simulink model "controller2"  (R2024b)
settings: Solver=FixedStepAuto  StartTime=0.0  StopTime=9  FixedStep=0.05  RelTol=1e-3
model workspace (MAT data in the model file):
  SamplePd = 0.05
values from neighbouring files (symbols this model uses):
  DryMass = 3    [FlightPathGeneration.m]
  LaunchSitePressure = PlanMeta(7)    [FlightAnalysis.m]    (also in FlightPathGeneration.m = 101325; TargetApogeeSelection.m = 101325)
  LaunchSiteTemperature = PlanMeta(6)    [FlightAnalysis.m]    (also in FlightPathGeneration.m = 288.15; TargetApogeeSelection.m = 288.15)
  MaximumDragArea = 0.01    [FlightPathGeneration.m]    (also in TargetApogeeSelection.m)
  MinimumDragArea = 0.0025    [FlightPathGeneration.m]    (also in TargetApogeeSelection.m)
  SimAngleSamples = linspace(0, pi/2, AngleSamples)    [FlightPathGeneration.m]
  SimGradAngleMesh = SimGradAngleMesh(end:-1:1, end:-1:1)'    [FlightPathGeneration.m]
  SimGradVMesh = SimGradVMesh(end:-1:1, end:-1:1)'    [FlightPathGeneration.m]
  SimMesh = centerPathAltitudes(end:-1:1, end:-1:1)'    [FlightPathGeneration.m]
  SimVelocitySamples = linspace(0, MaxVelocity, VelocitySamples)    [FlightPathGeneration.m]
undefined symbols (not defined in the file or in its folder): DiscIntNeverNeededParam
settings Model: Creator=natha  LastModifiedBy=natha

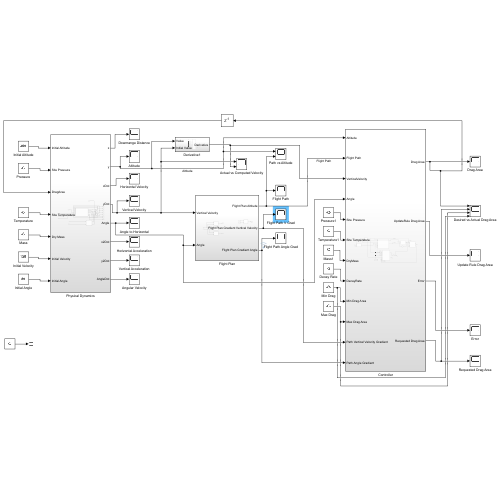
[thumbnail: Simulink's stored preview of the top-level diagram]
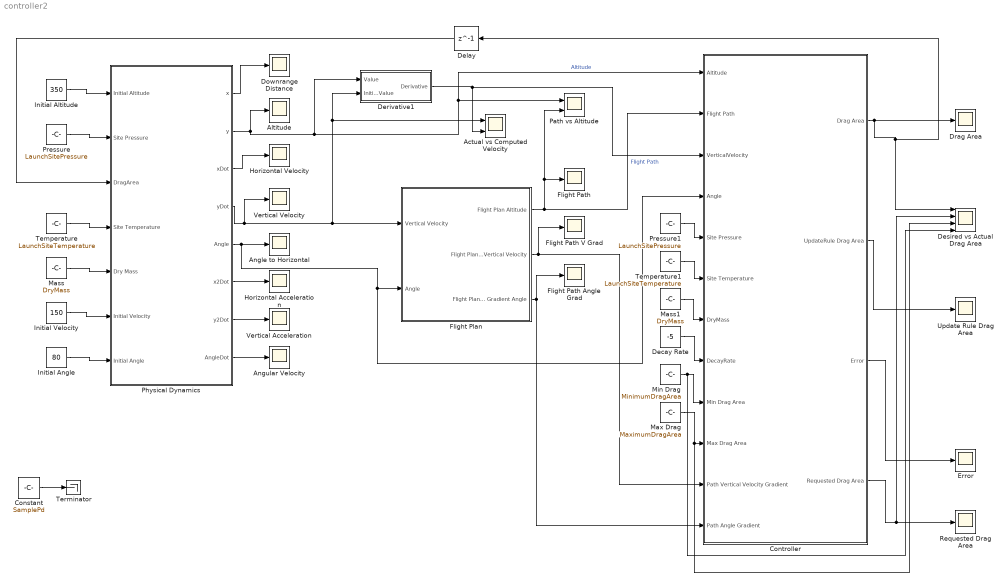
== system controller2 ==
  Actual vs Computed Velocity : Scope  NumInputPorts=2
  Altitude : Scope
  Angle to Horizontal : Scope
  Angular Velocity : Scope
  Constant : Constant  Value=SamplePd
  Controller : Subsystem
  Decay Rate : Constant  Value=-5
  Delay : Delay  DelayLength=1  InputProcessing=Columns as channels (frame based)
  Derivative1 : Subsystem
  Desired vs Actual Drag Area : Scope  NumInputPorts=4
  Downrange Distance : Scope
  Drag Area : Scope
  Error : Scope
  Flight Path : Scope
  Flight Path Angle Grad : Scope
  Flight Path V Grad : Scope
  Flight Plan : Subsystem
  Horizontal Acceleration : Scope
  Horizontal Velocity : Scope
  Initial Altitude : Constant  Value=350
  Initial Angle : Constant  Value=80
  Initial Velocity : Constant  Value=150
  Mass : Constant  Value=DryMass
  Mass1 : Constant  Value=DryMass
  Max Drag : Constant  Value=MaximumDragArea
  Min Drag : Constant  Value=MinimumDragArea
  Path vs Altitude : Scope  NumInputPorts=2
  Physical Dynamics : Subsystem
  Pressure : Constant  Value=LaunchSitePressure
  Pressure1 : Constant  Value=LaunchSitePressure
  Requested Drag Area : Scope
  Temperature : Constant  Value=LaunchSiteTemperature
  Temperature1 : Constant  Value=LaunchSiteTemperature
  Terminator : Terminator
  Update Rule Drag Area : Scope
  Vertical Acceleration : Scope
  Vertical Velocity : Scope
  wires:
  Initial Altitude/1 -> Physical Dynamics/1(Initial Altitude)
  Pressure/1 -> Physical Dynamics/2(Site Pressure)
  Temperature/1 -> Physical Dynamics/4(Site Temperature)
  Mass/1 -> Physical Dynamics/5(Dry Mass)
  Initial Velocity/1 -> Physical Dynamics/6(Initial Velocity)
  Initial Angle/1 -> Physical Dynamics/7(Initial Angle)
  Physical Dynamics/1(x) -> Downrange Distance/1
  Physical Dynamics/2(y) -> Derivative1/1(Value), Controller/1(Altitude), Path vs Altitude/1, Altitude/1  "Altitude"
  Physical Dynamics/3(xDot) -> Horizontal Velocity/1
  Physical Dynamics/4(yDot) -> Actual vs Computed Velocity/1, Derivative1/2(Initial Value), Flight Plan/1(Vertical Velocity), Vertical Velocity/1
  Physical Dynamics/5(Angle) -> Controller/4(Angle), Flight Plan/2(Angle), Angle to Horizontal/1
  Physical Dynamics/7(y2Dot) -> Vertical Acceleration/1
  Physical Dynamics/6(x2Dot) -> Horizontal Acceleration/1
  Flight Plan/1(Flight Plan Altitude) -> Controller/2(Flight Path), Path vs Altitude/2, Flight Path/1  "Flight Path"
  Flight Plan/2(Flight Plan Gradient Vertical Velocity) -> Controller/11(Path Vertical Velocity Gradient), Flight Path V Grad/1
  Flight Plan/3(Flight Plan Gradient Angle) -> Controller/12(Path Angle Gradient), Flight Path Angle Grad/1
  Min Drag/1 -> Desired vs Actual Drag Area/4, Controller/9(Min Drag Area)
  Max Drag/1 -> Desired vs Actual Drag Area/3, Controller/10(Max Drag Area)
  Decay Rate/1 -> Controller/8(DecayRate)
  Temperature1/1 -> Controller/6(Site Temperature)
  Pressure1/1 -> Controller/5(Site Pressure)
  Mass1/1 -> Controller/7(DryMass)
  Physical Dynamics/8(AngleDot) -> Angular Velocity/1
  Controller/2(UpdateRule Drag Area) -> Update Rule Drag Area/1
  Controller/1(Drag Area) -> Delay/1, Desired vs Actual Drag Area/1, Drag Area/1
  Controller/3(Error) -> Error/1
  Delay/1 -> Physical Dynamics/3(DragArea)
  Constant/1 -> Terminator/1
  Derivative1/1(Derivative) -> Controller/3(VerticalVelocity), Actual vs Computed Velocity/2
  Controller/4(Requested Drag Area) -> Desired vs Actual Drag Area/2, Requested Drag Area/1

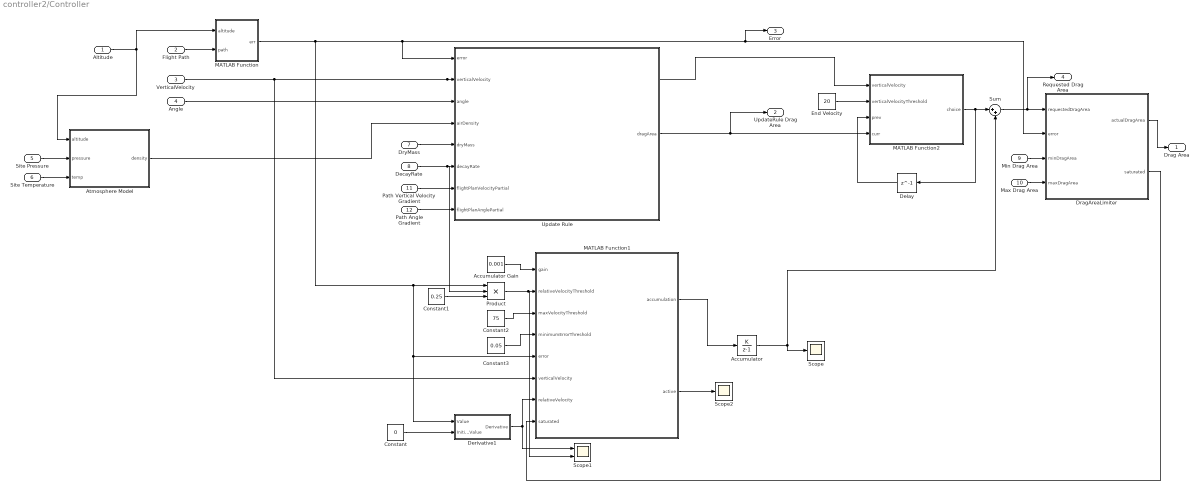
== system controller2/Controller ==
  Altitude : Inport
  Flight Path : Inport  Port=2
  VerticalVelocity : Inport  Port=3
  Angle : Inport  Port=4
  Site Pressure : Inport  Port=5
  Site Temperature : Inport  Port=6
  DryMass : Inport  Port=7
  DecayRate : Inport  Port=8
  Min Drag Area : Inport  Port=9
  Max Drag Area : Inport  Port=10
  Path Vertical Velocity Gradient : Inport  Port=11
  Path Angle Gradient : Inport  Port=12
  Accumulator : DiscreteIntegrator  IntegratorMethod=Accumulation: Forward Euler  SampleTime=-1  ICPrevOutput=DiscIntNeverNeededParam  ICPrevScaledInput=DiscIntNeverNeededParam
  Accumulator Gain : Constant  Value=0.001
  Atmosphere Model : MATLAB Function  TreatAsAtomicUnit=on
  Constant : Constant  Value=0
  Constant1 : Constant  Value=0.25
  Constant2 : Constant  Value=75
  Constant3 : Constant  Value=0.05
  Delay : Delay  DelayLength=1  InputProcessing=Columns as channels (frame based)
  Derivative1 : Subsystem
  DragAreaLimiter : MATLAB Function  TreatAsAtomicUnit=on
  End Velocity : Constant  Value=20
  MATLAB Function : MATLAB Function  TreatAsAtomicUnit=on
  MATLAB Function1 : MATLAB Function  TreatAsAtomicUnit=on
  MATLAB Function2 : MATLAB Function  TreatAsAtomicUnit=on
  Product : Product  Inputs=3
  Scope : Scope
  Scope1 : Scope  NumInputPorts=2
  Scope2 : Scope
  Sum : Sum  Inputs=|++
  Update Rule : MATLAB Function  TreatAsAtomicUnit=on
  Drag Area : Outport
  UpdateRule Drag Area : Outport  Port=2
  Error : Outport  Port=3
  Requested Drag Area : Outport  Port=4
  wires:
  DecayRate/1 -> Update Rule/6(decayRate), Product/2
  Max Drag Area/1 -> DragAreaLimiter/4(maxDragArea)
  DryMass/1 -> Update Rule/5(dryMass)
  Min Drag Area/1 -> DragAreaLimiter/3(minDragArea)
  Update Rule/1(dragArea) -> MATLAB Function2/4(curr), UpdateRule Drag Area/1
  Atmosphere Model/1(density) -> Update Rule/4(airDensity)
  Altitude/1 -> Atmosphere Model/1(altitude), MATLAB Function/1(altitude)
  MATLAB Function/1(err) -> Derivative1/1(Value), MATLAB Function1/5(error), Product/1, Update Rule/1(error), DragAreaLimiter/2(error), Error/1
  Site Temperature/1 -> Atmosphere Model/3(temp)
  Site Pressure/1 -> Atmosphere Model/2(pressure)
  Flight Path/1 -> MATLAB Function/2(path)
  Angle/1 -> Update Rule/3(angle)
  Path Angle Gradient/1 -> Update Rule/8(flightPlanAnglePartial)
  VerticalVelocity/1 -> MATLAB Function1/6(verticalVelocity), MATLAB Function2/1(verticalVelocity), Update Rule/2(verticalVelocity)
  Path Vertical Velocity Gradient/1 -> Update Rule/7(flightPlanVelocityPartial)
  MATLAB Function1/1(accumulation) -> Accumulator/1
  Accumulator Gain/1 -> MATLAB Function1/1(gain)
  Constant2/1 -> MATLAB Function1/3(maxVelocityThreshold)
  Constant3/1 -> MATLAB Function1/4(minimumErrorThreshold)
  Constant1/1 -> Product/3
  Product/1 -> Scope1/2, MATLAB Function1/2(relativeVelocityThreshold)
  Derivative1/1(Derivative) -> Scope1/1, MATLAB Function1/7(relativeVelocity)
  Constant/1 -> Derivative1/2(Initial Value)
  Accumulator/1 -> Sum/2, Scope/1
  MATLAB Function1/2(active) -> Scope2/1
  MATLAB Function2/1(choice) -> Sum/1, Delay/1
  Delay/1 -> MATLAB Function2/3(prev)
  End Velocity/1 -> MATLAB Function2/2(verticalVelocityThreshold)
  Sum/1 -> Requested Drag Area/1, DragAreaLimiter/1(requestedDragArea)
  DragAreaLimiter/1(actualDragArea) -> Drag Area/1
  DragAreaLimiter/2(saturated) -> MATLAB Function1/8(saturated)

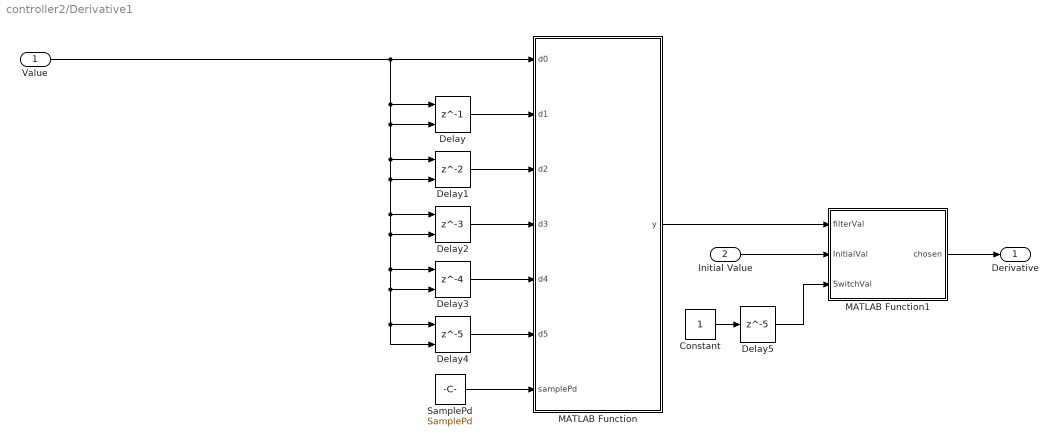
== system controller2/Derivative1 ==
  Value : Inport
  Initial Value : Inport  Port=2
  Constant : Constant
  Delay : Delay  DelayLength=1  InitialConditionSource=Input port  InputProcessing=Columns as channels (frame based)
      settings: InputPortMap=u0,p4
  Delay1 : Delay  InitialConditionSource=Input port  InputProcessing=Columns as channels (frame based)
      settings: InputPortMap=u0,p4
  Delay2 : Delay  DelayLength=3  InitialConditionSource=Input port  InputProcessing=Columns as channels (frame based)
      settings: InputPortMap=u0,p4
  Delay3 : Delay  DelayLength=4  InitialConditionSource=Input port  InputProcessing=Columns as channels (frame based)
      settings: InputPortMap=u0,p4
  Delay4 : Delay  DelayLength=5  InitialConditionSource=Input port  InputProcessing=Columns as channels (frame based)
      settings: InputPortMap=u0,p4
  Delay5 : Delay  DelayLength=5  InputProcessing=Columns as channels (frame based)
  MATLAB Function : MATLAB Function  TreatAsAtomicUnit=on
  MATLAB Function1 : MATLAB Function  TreatAsAtomicUnit=on
  SamplePd : Constant  Value=SamplePd
  Derivative : Outport
  wires:
  Value/1 -> Delay2/2, Delay3/2, Delay4/2, Delay4/1, Delay3/1, Delay2/1, Delay1/2, Delay1/1, Delay/2, Delay/1, MATLAB Function/1(d0)
  Delay/1 -> MATLAB Function/2(d1)
  Delay1/1 -> MATLAB Function/3(d2)
  Delay2/1 -> MATLAB Function/4(d3)
  Delay3/1 -> MATLAB Function/5(d4)
  Delay4/1 -> MATLAB Function/6(d5)
  SamplePd/1 -> MATLAB Function/7(samplePd)
  MATLAB Function1/1(chosen) -> Derivative/1
  MATLAB Function/1(y) -> MATLAB Function1/1(filterVal)
  Initial Value/1 -> MATLAB Function1/2(InitialVal)
  Delay5/1 -> MATLAB Function1/3(SwitchVal)
  Constant/1 -> Delay5/1

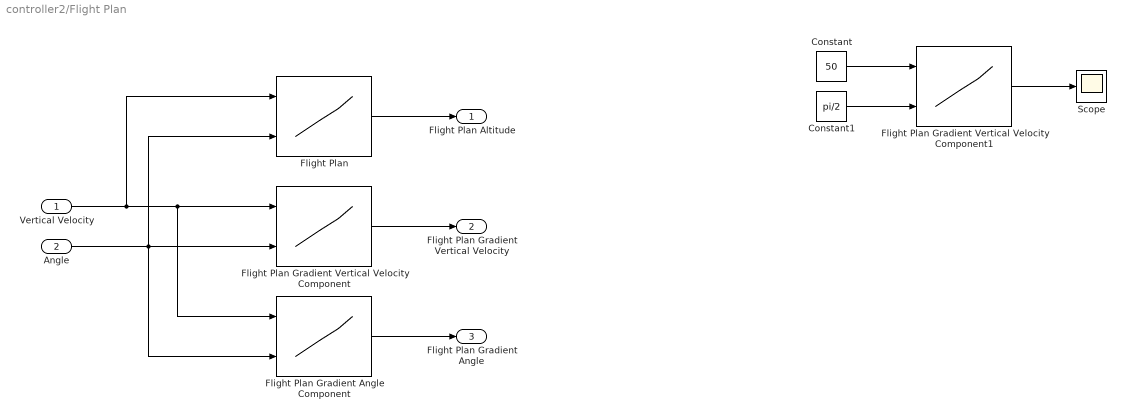
== system controller2/Flight Plan ==
  Vertical Velocity : Inport
  Angle : Inport  Port=2
  Constant : Constant  Value=50
  Constant1 : Constant  Value=pi/2
  Flight Plan : Lookup_n-D  BreakpointsForDimension1=SimVelocitySamples  BreakpointsForDimension2=SimAngleSamples  Table=SimMesh  InternalRulePriority=Speed  RndMeth=Simplest
      settings: InputPortMap=u0,u1
  Flight Plan Gradient Angle Component : Lookup_n-D  BreakpointsForDimension1=SimVelocitySamples  BreakpointsForDimension2=SimAngleSamples  Table=SimGradAngleMesh  InternalRulePriority=Speed  RndMeth=Simplest
      settings: InputPortMap=u0,u1
  Flight Plan Gradient Vertical Velocity Component : Lookup_n-D  BreakpointsForDimension1=SimVelocitySamples  BreakpointsForDimension2=SimAngleSamples  Table=SimGradVMesh  InternalRulePriority=Speed  RndMeth=Simplest
      settings: InputPortMap=u0,u1
  Flight Plan Gradient Vertical Velocity Component1 : Lookup_n-D  BreakpointsForDimension1=SimVelocitySamples  BreakpointsForDimension2=SimAngleSamples  Table=SimGradVMesh  InternalRulePriority=Speed  RndMeth=Simplest
      settings: InputPortMap=u0,u1
  Scope : Scope
  Flight Plan Altitude : Outport
  Flight Plan Gradient Vertical Velocity : Outport  Port=2
  Flight Plan Gradient Angle : Outport  Port=3
  wires:
  Flight Plan Gradient Vertical Velocity Component/1 -> Flight Plan Gradient Vertical Velocity/1
  Angle/1 -> Flight Plan Gradient Angle Component/2, Flight Plan Gradient Vertical Velocity Component/2, Flight Plan/2
  Vertical Velocity/1 -> Flight Plan Gradient Angle Component/1, Flight Plan Gradient Vertical Velocity Component/1, Flight Plan/1
  Flight Plan Gradient Angle Component/1 -> Flight Plan Gradient Angle/1
  Flight Plan/1 -> Flight Plan Altitude/1
  Constant1/1 -> Flight Plan Gradient Vertical Velocity Component1/2
  Constant/1 -> Flight Plan Gradient Vertical Velocity Component1/1
  Flight Plan Gradient Vertical Velocity Component1/1 -> Scope/1

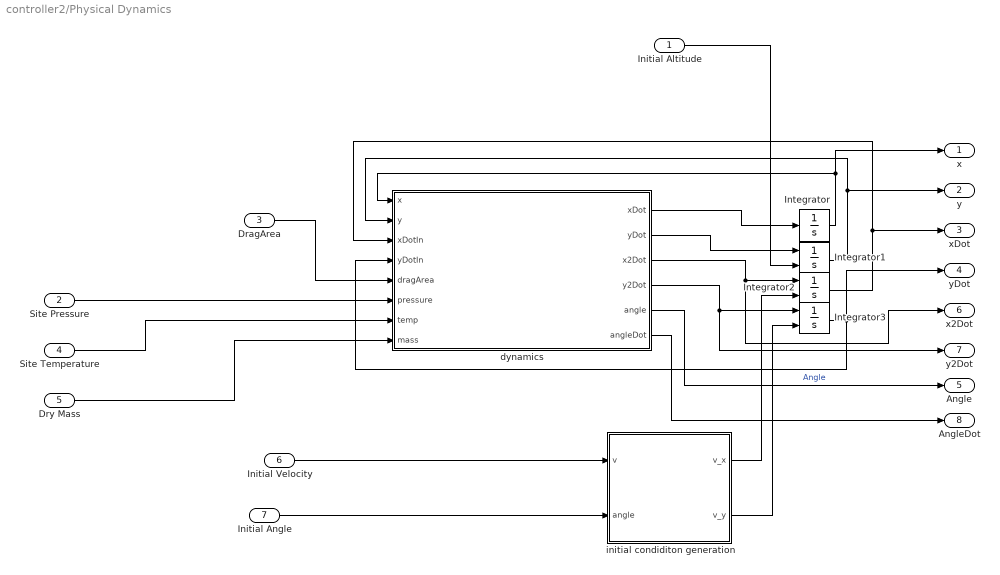
== system controller2/Physical Dynamics ==
  Initial Altitude : Inport
  Site Pressure : Inport  Port=2
  DragArea : Inport  Port=3
  Site Temperature : Inport  Port=4
  Dry Mass : Inport  Port=5
  Initial Velocity : Inport  Port=6
  Initial Angle : Inport  Port=7
  Integrator : Integrator
  Integrator1 : Integrator  InitialConditionSource=external
  Integrator2 : Integrator  InitialConditionSource=external
  Integrator3 : Integrator  InitialConditionSource=external
  dynamics : MATLAB Function  TreatAsAtomicUnit=on
  initial condiditon generation : MATLAB Function  TreatAsAtomicUnit=on
  x : Outport
  y : Outport  Port=2
  xDot : Outport  Port=3
  yDot : Outport  Port=4
  Angle : Outport  Port=5
  x2Dot : Outport  Port=6
  y2Dot : Outport  Port=7
  AngleDot : Outport  Port=8
  wires:
  dynamics/1(xDot) -> Integrator/1
  Integrator2/1 -> dynamics/3(xDotIn), xDot/1
  dynamics/4(y2Dot) -> y2Dot/1, Integrator3/1
  dynamics/5(angle) -> Angle/1  "Angle"
  dynamics/2(yDot) -> Integrator1/1
  initial condiditon generation/2(v_y) -> Integrator3/2
  dynamics/3(x2Dot) -> x2Dot/1, Integrator2/1
  initial condiditon generation/1(v_x) -> Integrator2/2
  DragArea/1 -> dynamics/5(dragArea)
  Integrator3/1 -> dynamics/4(yDotIn), yDot/1
  Integrator/1 -> x/1, dynamics/1(x)
  Integrator1/1 -> y/1, dynamics/2(y)
  Dry Mass/1 -> dynamics/8(mass)
  Site Pressure/1 -> dynamics/6(pressure)
  Initial Angle/1 -> initial condiditon generation/2(angle)
  Initial Altitude/1 -> Integrator1/2
  Site Temperature/1 -> dynamics/7(temp)
  Initial Velocity/1 -> initial condiditon generation/1(v)
  dynamics/6(angleDot) -> AngleDot/1

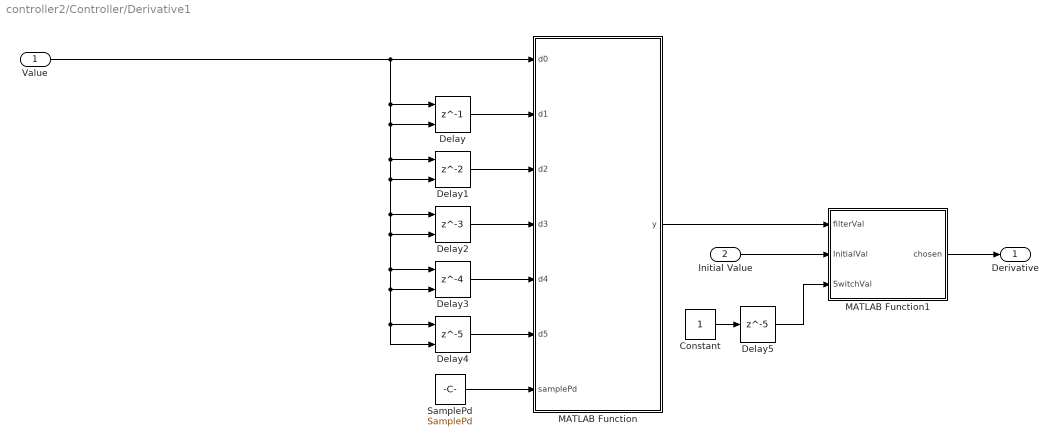
== system controller2/Controller/Derivative1 ==
  Value : Inport
  Initial Value : Inport  Port=2
  Constant : Constant
  Delay : Delay  DelayLength=1  InitialConditionSource=Input port  InputProcessing=Columns as channels (frame based)
      settings: InputPortMap=u0,p4
  Delay1 : Delay  InitialConditionSource=Input port  InputProcessing=Columns as channels (frame based)
      settings: InputPortMap=u0,p4
  Delay2 : Delay  DelayLength=3  InitialConditionSource=Input port  InputProcessing=Columns as channels (frame based)
      settings: InputPortMap=u0,p4
  Delay3 : Delay  DelayLength=4  InitialConditionSource=Input port  InputProcessing=Columns as channels (frame based)
      settings: InputPortMap=u0,p4
  Delay4 : Delay  DelayLength=5  InitialConditionSource=Input port  InputProcessing=Columns as channels (frame based)
      settings: InputPortMap=u0,p4
  Delay5 : Delay  DelayLength=5  InputProcessing=Columns as channels (frame based)
  MATLAB Function : MATLAB Function  TreatAsAtomicUnit=on
  MATLAB Function1 : MATLAB Function  TreatAsAtomicUnit=on
  SamplePd : Constant  Value=SamplePd
  Derivative : Outport
  wires:
  Value/1 -> Delay2/2, Delay3/2, Delay4/2, Delay4/1, Delay3/1, Delay2/1, Delay1/2, Delay1/1, Delay/2, Delay/1, MATLAB Function/1(d0)
  Delay/1 -> MATLAB Function/2(d1)
  Delay1/1 -> MATLAB Function/3(d2)
  Delay2/1 -> MATLAB Function/4(d3)
  Delay3/1 -> MATLAB Function/5(d4)
  Delay4/1 -> MATLAB Function/6(d5)
  SamplePd/1 -> MATLAB Function/7(samplePd)
  MATLAB Function1/1(chosen) -> Derivative/1
  MATLAB Function/1(y) -> MATLAB Function1/1(filterVal)
  Initial Value/1 -> MATLAB Function1/2(InitialVal)
  Delay5/1 -> MATLAB Function1/3(SwitchVal)
  Constant/1 -> Delay5/1

== matlab function controller2/Derivative1/MATLAB Function ==
  data: d0 input; y output; d1 input; d2 input; d3 input; d4 input; d5 input; samplePd input
function y = fcn(d0, d1, d2, d3, d4, d5, samplePd)
y = (d0 + 3*d1 + 2*d2 - 2*d3 - 3*d4 -d5)/16/samplePd;
end

== matlab function controller2/Controller/Derivative1/MATLAB Function ==
  data: d0 input; y output; d1 input; d2 input; d3 input; d4 input; d5 input; samplePd input
function y = fcn(d0, d1, d2, d3, d4, d5, samplePd)
y = (d0 + 3*d1 + 2*d2 - 2*d3 - 3*d4 -d5)/16/samplePd;
end

== matlab function controller2/Controller/Derivative1/MATLAB Function1 ==
  data: filterVal input; chosen output; InitialVal input; SwitchVal input
function chosen = loadSwitch(filterVal, InitialVal, SwitchVal)
if(SwitchVal ~= 0)
    chosen = filterVal;
else
    chosen = InitialVal;
end
end

== matlab function controller2/Controller/MATLAB Function2 ==
  data: verticalVelocity input; choice output; verticalVelocityThreshold input; prev input; curr input
function choice = clamp(verticalVelocity, verticalVelocityThreshold, prev, curr)
if(verticalVelocity < verticalVelocityThreshold)
    choice = prev;
else
    choice = curr;
end

== matlab function controller2/Derivative1/MATLAB Function1 ==
  data: filterVal input; chosen output; InitialVal input; SwitchVal input
function chosen = loadSwitch(filterVal, InitialVal, SwitchVal)
if(SwitchVal ~= 0)
    chosen = filterVal;
else
    chosen = InitialVal;
end
end

== matlab function controller2/Physical Dynamics/initial condiditon generation ==
  data: v input; v_x output; angle input; v_y output
function [v_x, v_y] = initialConditions(v, angle)
v_x = v * cos(angle * pi / 180);
v_y = v * sin(angle * pi / 180);
end

== matlab function controller2/Physical Dynamics/dynamics ==
  data: xDot output; yDot output; x2Dot output; y2Dot output; x input; y input; xDotIn input; yDotIn input; dragArea input; angle output; pressure input; temp input; mass input; angleDot output
function [xDot,yDot, x2Dot, y2Dot, angle, angleDot] = dynamics(x, y, xDotIn, yDotIn, dragArea, pressure, temp, mass)
%constants---
g = 9.8;
%------------
x;
xDot = xDotIn;
yDot = yDotIn;
x2Dot = -1/2/mass * densityFromAltitude(y, pressure, temp) * dragArea * sqrt(xDot * xDot + yDot * yDot) * xDot;
y2Dot = -1/2/mass * densityFromAltitude(y, pressure, temp) * dragArea * sqrt(xDot * xDot + yDot * yDot) * yDot - g;
angle = atan(yDot/xDot);
angleDot = (y2Dot * xDot - yDot * x2Dot) / (xDot * xDot + yDot * yDot);
end


function density = densityFromAltitude(altitude, p0, T0)
    % Constants
    L = 0.0065;      % K/m temperature lapse rate
    g = 9.80665;     % m/s^2 gravitational constant
    R = 8.31446;     % J/(mol*K) Ideal gas constant
    M = 0.0289652;   % kg/mol Molar mass of air
    density = p0*M/(R*T0)*(1-L*altitude/T0).^(g*M/(R*L)-1);
end

== matlab function controller2/Controller/Update Rule ==
  data: error input; dragArea output; verticalVelocity input; angle input; airDensity input; dryMass input; decayRate input; flightPlanVelocityPartial input; flightPlanAnglePartial input
function dragArea = updateRule(error, verticalVelocity, angle, airDensity, dryMass, decayRate, flightPlanVelocityPartial, flightPlanAnglePartial)
g = 9.8;
dragArea = 2 * dryMass * sin(angle) * (decayRate * error - verticalVelocity - g * (flightPlanVelocityPartial + flightPlanAnglePartial * sin(2*angle) / (2 * verticalVelocity))) / (airDensity * verticalVelocity * verticalVelocity * flightPlanVelocityPartial);
end

== matlab function controller2/Controller/Atmosphere Model ==
  data: density output; altitude input; pressure input; temp input
function density = airDensity(altitude, pressure, temp)
    % Constants
    L = 0.0065;      % K/m temperature lapse rate
    g = 9.80665;     % m/s^2 gravitational constant
    R = 8.31446;     % J/(mol*K) Ideal gas constant
    M = 0.0289652;   % kg/mol Molar mass of air
    density = pressure*M/(R*temp)*(1-L*altitude/temp).^(g*M/(R*L)-1);
end

== matlab function controller2/Controller/DragAreaLimiter ==
  data: requestedDragArea input; actualDragArea output; error input; minDragArea input; maxDragArea input; saturated output
function [actualDragArea, saturated] = dragLimit(requestedDragArea, error, minDragArea, maxDragArea)
        if( requestedDragArea < maxDragArea && requestedDragArea > minDragArea)
            actualDragArea = requestedDragArea;
            saturated = 0;
        else
            saturated = 1;
            if(error > 0) 
                actualDragArea = maxDragArea;
            else
                actualDragArea = minDragArea;
            end
        end
end

== matlab function controller2/Controller/MATLAB Function ==
  data: altitude input; err output; path input
function err = error(altitude, path)
err = altitude - path;
end

== matlab function controller2/Controller/MATLAB Function1 ==
  data: gain input; accumulation output; relativeVelocityThreshold input; maxVelocityThreshold input; minimumErrorThreshold input; error input; verticalVelocity input; relativeVelocity input; active output; saturated input
function [accumulation, active] = accumulationInput(gain, relativeVelocityThreshold, maxVelocityThreshold, minimumErrorThreshold, error, verticalVelocity, relativeVelocity, saturated)
    active = isBadApproach(relativeVelocity, relativeVelocityThreshold, error, minimumErrorThreshold, verticalVelocity, maxVelocityThreshold);
    if(active == 0 && saturated == 0)
        accumulation = gain * error;
    else 
        accumulation = 0;
    end
end

function condition = isBadApproach(relativeVelocity, relativeVelocityThreshold, error, errorThreshold, verticalVelocity, verticalVelocityThreshold)
    if(abs(error) < errorThreshold || verticalVelocity > verticalVelocityThreshold)
        condition = 1;
    else
        if(relativeVelocityThreshold > 0)
            if(relativeVelocity < relativeVelocityThreshold)
                condition = 0;
            else
                condition = 2;
            end
        else
            if(relativeVelocity > relativeVelocityThreshold)
                condition = 0;
            else
                condition = 3;
            end
        end
    end
end
